simulink model "OneTwoTwo_Two"  (R2022b)
settings: Solver=VariableStepAuto  StartTime=0.0  StopTime=2  RelTol=1e-3
libraries: simulink x1
settings Model: Creator=yeyi5  LastModifiedBy=yeyi5

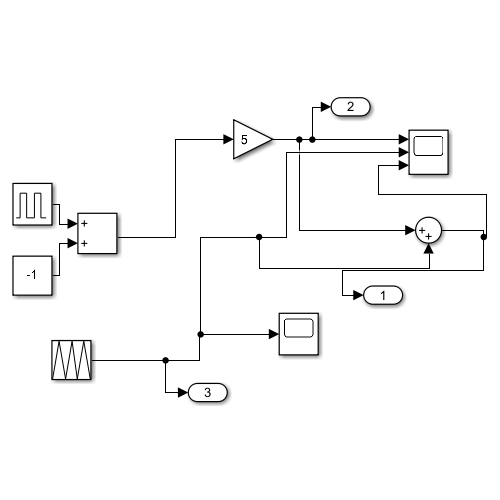
[thumbnail: Simulink's stored preview of the top-level diagram]
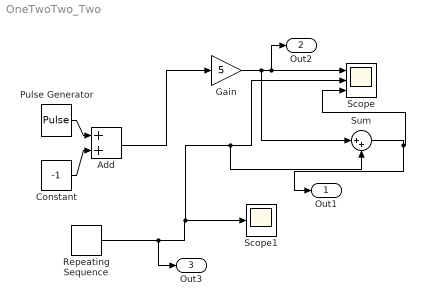
== system OneTwoTwo_Two ==
  Add : Sum
  Constant : Constant  Value=-1
  Gain : Gain  Gain=5
  Pulse Generator : DiscretePulseGenerator  PulseType=Time based  Amplitude=2  Period=1/5  PulseWidth=50
  Repeating Sequence : simulink/Sources/Repeating Sequence  rep_seq_t=[0, 0.1, 0.2]  rep_seq_y=[-5, 5, -5]
  Scope : Scope  NumInputPorts=3
  Scope1 : Scope
  Sum : Sum  Inputs=|++
  Out1 : Outport
  Out2 : Outport  Port=2
  Out3 : Outport  Port=3
  wires:
  Pulse Generator/1 -> Add/1
  Constant/1 -> Add/2
  Add/1 -> Gain/1
  Gain/1 -> Sum/1, Out2/1, Scope/1
  Repeating Sequence/1 -> Out3/1, Sum/2, Scope/2, Scope1/1
  Sum/1 -> Out1/1, Scope/3
